simulink model "ref3sa_template"  (Simulink 4.00)
settings: Solver=FixedStepDiscrete  StartTime=0.0  StopTime=60  FixedStep=.0005  RelTol=1e-3
settings Model: Creator=root  LastModifiedBy=root  LimitDataPoints=off  ExtModeTrigMode=oneshot  ExtModeArmWhenConnect=off  ExtModeAutoUpdateStatusClock=off

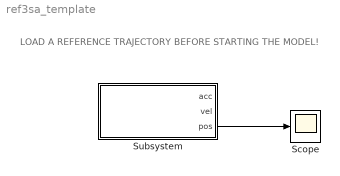
== system ref3sa_template ==
  note: LOAD A REFERENCE TRAJECTORY BEFORE STARTING THE MODEL!
  Scope : Scope
      settings: TimeRange=60  YMin=-0.1  YMax=1  SaveToWorkspace=off  SaveName=ScopeData  LimitDataPoints=on  MaxDataPoints=5000
  Subsystem : Subsystem
      settings: OpenFcn=cb_axes 1  RTWFcnNameOpts=Auto  RTWFileNameOpts=Auto
      mask Type: Ref3
      mask Display: disp('Ref3');
  wires:
  Subsystem/3(pos) -> Scope/1

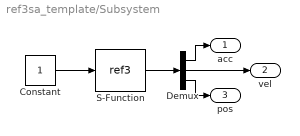
== system ref3sa_template/Subsystem ==
  Constant : Constant  Value=1
  Demux : Demux  Outputs=3  BusSelectionMode=off
  S-Function : S-Function  FunctionName=ref3  Parameters=ref_part  PortCounts=[]  SFunctionModules=''
      settings: OpenFcn=global ref_part; r3g_main
  acc : Outport  Port=1
  vel : Outport  Port=2
  pos : Outport  Port=3
  wires:
  Constant/1 -> S-Function/1
  S-Function/1 -> Demux/1
  Demux/1 -> acc/1
  Demux/2 -> vel/1
  Demux/3 -> pos/1
